simulink model "bus_roadtest_v3"  (R2018a)
settings: Solver=ode3  StartTime=0.0  StopTime=inf  FixedStep=0.01  RelTol=1e-3  EnableMultiTasking=on
PostLoadFcn:
  | , if any(exist('dsrtsu_mdlpostloadfcn', 'file') == [2, 3, 6]), try dsrtsu_mdlpostloadfcn('Execute', bdroot); catch fprintf('Error in PostLoadFcn (dsrtsu_mdlpostloadfcn) for model "%s":\n %s\n', bdroot, lasterr); end, end,
InitFcn:
  | bus_roadtest_v3_initial
values from neighbouring files (symbols this model uses):
  ay_max = 2    [Ini.m]
  delta_t = 0.01    [Ini.m]
  end_left_pass = 1    [Ini.m]
  end_right_pass = 0    [Ini.m]
  finish_node_id = length(Map_data(:,1))    [Ini.m]
  forward_length = 15    [Ini.m]
  gamma = sqrt(N_xaug+lambda)    [bus_roadtest_v3_initial.m]
  k_safe = 1    [Ini.m]
  nodes = nodes(1:index_node,:)    [Ini.m]
  rmin = 10    [Ini.m]
  segments = zeros(length(xy_ends_Pos(:,1)),3)    [Ini.m]
  start_node_id = 1    [Ini.m]
  Ts = 0.01    [bus_roadtest_v3_initial.m]
  Veh_CG = [0.5, 0.2]    [Ini.m]
  Veh_size = [1.99986,6.09558]    [Ini.m]
  vmax = 6    [Ini.m]
  weight = [weight_0,weight_0_cov,weight_i]    [bus_roadtest_v3_initial.m]
undefined symbols (not defined in the file or in its folder): Brake_table, DiscIntNeverNeededParam, Map_data, R, REF_GPS_RFS, Steer_gain_table, T
libraries: rtican x71, simulink x26, rti1401lib_adc_type4 x8, rti1401lib_dio_type4 x1
(part 15 of 18)

== matlab function bus_roadtest_v3/Positioning_module/ITRI_MM/UKF_Only/GNSS_UKF_MM ==
  data: seg_id_near output; Map_data input; dist_op output; Position_X input; op_distance output; Oi_near output; num_lane_direction output; seg_heading output; seg_LaneWidth output; Postion_Y input; Position_H input
function [seg_id_near,dist_op,op_distance,Oi_near,num_lane_direction,seg_heading,seg_LaneWidth]= fcn(Map_data,Position_X,Postion_Y,Position_H)

%%% Map_data=[Seg_XY SLOPE_SEG SHIFT_SEG Heading_X LENGTH_SEG]; nx8
XY_ID=Map_data(:,1);
XY_INI=Map_data(:,2:3);
XY_END=Map_data(:,4:5);
SLOPE_SEG=Map_data(:,6);
SHIFT_SEG=Map_data(:,7);
HEADING_DIFFERENCE_VEH_ROAD = 45*pi/180;
DIST_THREAD_5 = 4;

m=length(XY_ID);
oi_xy=zeros(m,2);
dist_op=zeros(m,1);
for i =1:m
    if SLOPE_SEG(i) == inf
        oi_xy(i,1) = XY_INI(i,1); % x position of the projection point on this segment
        oi_xy(i,2) = Postion_Y;
    elseif SLOPE_SEG(i)==0
        oi_xy(i,1) = Position_X;
        oi_xy(i,2) = XY_INI(i,2);
    else
        a_j = -1/SLOPE_SEG(i);
        b_j = Postion_Y - a_j*Position_X;
        oi_xy(i,1) = (b_j-SHIFT_SEG(i))/(SLOPE_SEG(i)-a_j); % x position of the i-th projection point
        oi_xy(i,2) = (SLOPE_SEG(i)*b_j - a_j*SHIFT_SEG(i))/(SLOPE_SEG(i)-a_j); % y position of the i-th projection point 
    end          
end

for i = 1:length(oi_xy(:,1));
    dist_op(i,1)=sqrt((oi_xy(i,1)-Position_X)^2+(oi_xy(i,2)-Postion_Y)^2);     
end

[seg_id_near,op_distance,oi_near,note,seg_direction,head_err,num_lane_direction,seg_heading] = MM(Position_H*180/pi,[Position_X;Postion_Y],oi_xy,dist_op,Map_data,HEADING_DIFFERENCE_VEH_ROAD,DIST_THREAD_5);
Oi_near=oi_near';
[~,seg_id_ind] = max(XY_ID == seg_id_near);
seg_LaneWidth = Map_data(seg_id_ind,11);
seg_Curvature = Map_data(seg_id_ind,14);

%% MM function
function [seg_id_near,op_distance,oi_near,note,seg_direction,head_err,num_lane_direction,seg_heading] = MM(heading,X_pos,oi_xy,dist_op,Map_data,HEADING_DIFFERENCE_VEH_ROAD,DIST_THREAD_5)
note=0;
seg_id_near=double(0);
op_distance=0;
oi_near=zeros(1,2);
end_pt=zeros(1,2);
seg_direction=0;
[dist_sort,index] = sort(dist_op);
index=[index,zeros(length(index),1)];

xy_ini = Map_data(:,2:3);
xy_end = Map_data(:,4:5);
SLOPE_SEG = Map_data(:,6);
seg_id = Map_data(:,1);
LENGTH_SEG = Map_data(:,9);
SEG_GPS_HEAD = Map_data(:,8);
SEG_GPS_HEAD=[seg_id SEG_GPS_HEAD];

%%    Map Matching

for j = 1:length(xy_ini(:,1));
    i = index(j,1);
    dis_temp1 = sqrt((xy_ini(i,1)-oi_xy(i,1))^2+(xy_ini(i,2)-oi_xy(i,2))^2);
    dis_temp2 = sqrt((xy_end(i,1)-oi_xy(i,1))^2+(xy_end(i,2)-oi_xy(i,2))^2);
 
    if (dis_temp1 <= LENGTH_SEG(i)&& dis_temp2 <= LENGTH_SEG(i));
        index(j,2) = 1; %oi_xy lies in between xy_ini and xy_end
    else index(j,2) = 0;
    end
end

%"possible_seg" contains the sequence of possible segment index
ind_temp = find(index(1:end,2)==1);
% ind_temp=ind_temp(1);
if isempty(ind_temp);
   note = 1;  % 1: the projection point is not between two segment ends for any road segment;
              % search nearest segment by finding the nearest segment end!             
   %compare distances between ends and X_pos!     
    dist_ini = rel_dist_xy(X_pos,xy_ini);
    dist_end = rel_dist_xy(X_pos,xy_end);
  
    [min_dis_ini,junk1] = min(dist_ini);   %-------------------------------------------------哪來的junk 1 &2 ?
    [min_dis_end,junk2] = min(dist_end);
    if min_dis_ini<= min_dis_end; %X_pos is closer to the end
       possible_seg = junk1; %index
       end_pt = xy_ini(junk1,1:end);
    else 
       possible_seg = junk2; %index
       end_pt = xy_end(junk2,1:end);
    end

    seg_id_near = seg_id(possible_seg);
    
    op_distance = dist_op(possible_seg);
    oi_near = oi_xy(possible_seg,1:2);
    if possible_seg>1 && possible_seg<length(seg_id)
    op_distance_n=rel_dist_xy(X_pos,oi_near);
    min_ini_pos=rel_dist_xy(X_pos,xy_ini(possible_seg,:));
    min_end_pos=rel_dist_xy(X_pos,xy_end(possible_seg,:));
    if op_distance_n<min_ini_pos && op_distance_n<min_end_pos
        note = 0;
    else
        note = 1;
    end
    else
        op_distance_n=rel_dist_xy(X_pos,oi_near);
        min_ini_pos=rel_dist_xy(X_pos,xy_ini(possible_seg,:));
        min_end_pos=rel_dist_xy(X_pos,xy_end(possible_seg,:));
    end
    
%    seg_direction = Get_Seg_Heading(seg_id_near,heading);
%    %%%不用老師程式--
    temp_ind = find(SEG_GPS_HEAD(:,1) == seg_id_near);
    head_err = abs(heading-SEG_GPS_HEAD(temp_ind(1),2)); 
    if head_err <= HEADING_DIFFERENCE_VEH_ROAD
    seg_direction = 1; %1= along slope, 2:adverse
    elseif head_err>=HEADING_DIFFERENCE_VEH_ROAD && head_err<=90
    seg_direction = 0; %unknown
    else
    seg_direction = 2;
    end
%     %%%不用老師程式--
 elseif length(ind_temp(1)) ==1; %only 
%      find one segment candidate
       note = 0; % 0: the projection point lies between two ends of each segment    
       possible_seg = index(ind_temp(1),1);
       seg_id_near = seg_id(possible_seg);
       op_distance = dist_op(possible_seg);
       oi_near = oi_xy(possible_seg,1:2);
       end_pt = [0,0]; % temp./unused nominal values
%      seg_direction = Get_Seg_Heading(seg_id_near,heading); %get road segment heading direction

        temp_ind = find(SEG_GPS_HEAD(:,1) == seg_id_near);
        head_err = abs(heading-SEG_GPS_HEAD(temp_ind(1),2)); 
       if head_err <= HEADING_DIFFERENCE_VEH_ROAD;
            seg_direction = 1; %1= along slope, 2:adverse
       elseif head_err>=HEADING_DIFFERENCE_VEH_ROAD && head_err<=90
            seg_direction = 0; %unknown
       else
            seg_direction = 2;
       end
       %Now compare the distances between X_pos and all segment ends with
       %op_distance. If find closer node, may discard previous found segment.
       
       dist_ini = rel_dist_xy(X_pos,xy_ini);
       dist_end = rel_dist_xy(X_pos,xy_end);
           %dis_min = min(dist_ini,dist_end);
           %dis_min_val = min(dis_min);
           %temp_a = find(dis_min == dis_min_val); % diff, segments may have the same node!
       [min_dis_ini,junk1] = min(dist_ini);
       [min_dis_end,junk2] = min(dist_end);
       dis_min_val = min(min_dis_ini,min_dis_end);
       
    if dis_min_val < op_distance;%min(op_distance); %X_pos is closer to one of the segment ends than its project point         
       note = 2; %Change the "note" value! 
                 %special case: the found projection pt. (oi_near) lie(s) between two ends 
                 %of one segment, but the associated segments may not
                 %the nearest road segments.          
       %search the nearest node of road segments. 
        if min_dis_ini<= min_dis_end;
           temp_a = junk1;
           end_pt = xy_ini(junk1,1:end);
        else 
           temp_a = junk2;
           end_pt = xy_end(junk2,1:end);
        end
       
        
        if length(temp_a)>1; %multiple segment case
            
           seg_head_pos = SEG_GPS_HEAD(temp_a,2); %road segment heading in the positive slope direction
%            seg_head_neg = SEG_GPS_HEAD(temp_a,3);
           
           %find smallest heading discrepancy in positive slope direction
           [junk1,ind_pos] = min(abs(heading - seg_head_pos(1:end)));
               
           %find smallest heading discrepancy in negative/adverse slope direction
%            [junk2,ind_neg] = min(abs(angle_convert(heading - seg_head_neg(1:end))));
           
           %compare two smallest heading erros of two adverse directions
 
              ind = temp_a(ind_pos);
              seg_id_near = seg_id(ind);
              op_distance = dist_op(ind);
              oi_near = oi_xy(ind,1:2);
              temp_ind = find(SEG_GPS_HEAD(:,1) == seg_id_near);
              head_err = abs(heading-SEG_GPS_HEAD(temp_ind(1),2)); 

              if head_err <= HEADING_DIFFERENCE_VEH_ROAD;
                    seg_direction = 1; %1= along slope, 2:adverse
              elseif head_err>=HEADING_DIFFERENCE_VEH_ROAD && head_err<=90
                    seg_direction = 0; %unknown
              else
                    seg_direction = 2;
              end
       
        else %single segment case
              temp_ind = find(SEG_GPS_HEAD(:,1) == seg_id_near);
              head_err = abs(heading-SEG_GPS_HEAD(temp_ind(1),2)); 

              if head_err <= HEADING_DIFFERENCE_VEH_ROAD;
                    seg_direction = 1; %1= along slope, 2:adverse
              elseif head_err>=HEADING_DIFFERENCE_VEH_ROAD && head_err<=90
                    seg_direction = 0; %unknown
              else
                    seg_direction = 2;
              end
                 seg_id_near = seg_id(temp_a);
                 op_distance = dist_op(temp_a);
                 oi_near = oi_xy(temp_a,1:2);
        end
    end
 else %multiple segment candidates
       note = 0; % 0: the projection point lies between two ends of each segment          
       cand_seg = index(ind_temp,1);
       %cand_id = seg_id(cand_seg(1:2)); % only check the first two colsest segment candidate
       cand_op_dist = dist_op(cand_seg(1:2));
       
       %find road heading for the first two candidates
        head_pos = SEG_GPS_HEAD(cand_seg(1:2),2);

       %first candidate
        err_1 =  abs(heading - head_pos(1));
        %temp = [head_pos(1),head_neg(1)];
        %cand_head(1) = temp(ii);
        %clear ii;
       %second candidate
        err_2 = abs(heading - head_pos(2));
        %temp = [head_pos(2),head_neg(2)];
        %cand_head(2) = temp(ii);
        %clear ii;
        
       %compare two heading errors
        if err_1<= err_2 && err_1< HEADING_DIFFERENCE_VEH_ROAD; % HEADING_DIFFERENCE_VEH_ROAD = 45/180*pi
           possible_seg =  cand_seg(1);
           seg_direction = 1;
        elseif err_2< err_1 && ((cand_op_dist(2)-cand_op_dist(1))< DIST_THREAD_5); %DIST_THREAD_5 = 9 m
           possible_seg = cand_seg(2); 
           seg_direction = 2;
        else
           possible_seg = cand_seg(1);
           seg_direction = 1;
        end
        
       clear err_1 err_2 cand_op_dist cand_seg head_pos head_neg direction_1 direction_2;
       %possible_seg = index(ind_temp,1);       
       seg_id_near = seg_id(possible_seg);
       op_distance = dist_op(possible_seg);
       oi_near = oi_xy(possible_seg,1:2);
       end_pt = [0,0]; % temp./unused nominal values
        
       %Now compare the distances between X_pos and all segment ends with
       %above op_distance.
       %compute distances between X_pos and all segment ends
       dist_ini = rel_dist_xy(X_pos,xy_ini);
       dist_end = rel_dist_xy(X_pos,xy_end);
           %dis_min = min(dist_ini,dist_end);
           %dis_min_val = min(dis_min);
           %temp_a = find(dis_min == dis_min_val); % diff, segments may have the same node!
       [min_dis_ini,junk1] = min(dist_ini);
       [min_dis_end,junk2] = min(dist_end);
       dis_min_val = min(min_dis_ini,min_dis_end); 
       
    if dis_min_val < op_distance; %min(op_distance); %X_pos is closer to one of the segment ends than its project point         
       note = 2; %Change the note value! 
                 %special case: the found projection pt. (oi_near) lie(s) between two ends 
                 %of one segment, but the associated segments may not be
                 %the nearest road segments.          
       %search the nearest node of road segments. 
        if min_dis_ini<= min_dis_end;
           temp_a = junk1;
           end_pt = xy_ini(junk1,1:2);
        else 
           temp_a = junk2;
           end_pt = xy_end(junk2,1:2);
        end
        clear junk1 junk2;
        
        if length(temp_a)>1; %multiple segment case, then compare heading with road segment heading
          
           seg_head_pos = SEG_GPS_HEAD(temp_a,2);
           [junk1,ind_pos] = min(abs(heading - seg_head_pos(1:end)));


              ind = temp_a(ind_pos);
              seg_id_near = seg_id(ind);
              op_distance = dist_op(ind);
              oi_near = oi_xy(ind,1:2);

              temp_ind = find(SEG_GPS_HEAD(:,1) == seg_id_near);
              head_err = abs(heading-SEG_GPS_HEAD(temp_ind(1),2)); 

              if head_err <= HEADING_DIFFERENCE_VEH_ROAD;
                    seg_direction = 1; %1= along slope, 2:adverse
              elseif head_err>=HEADING_DIFFERENCE_VEH_ROAD && head_err<=90
                    seg_direction = 0; %unknown
              else
                    seg_direction = 2;
              end

       
        else %determine road direction is positive or negative slope direction

             seg_id_near = seg_id(temp_a);
             op_distance = dist_op(temp_a);
             oi_near = oi_xy(temp_a,1:2);
             temp_ind = find(SEG_GPS_HEAD(:,1) == seg_id_near);
              head_err = abs(heading-SEG_GPS_HEAD(temp_ind(1),2)); 

              if head_err <= HEADING_DIFFERENCE_VEH_ROAD;
                    seg_direction = 1; %1= along slope, 2:adverse
              elseif head_err>=HEADING_DIFFERENCE_VEH_ROAD && head_err<=90
                    seg_direction = 0; %unknown
              else
                    seg_direction = 2;
              end

        end
    end
           
end
%% check projection distance positive or negative Y=AX+B ;AX+B-Y>0 or AX+B-Y<0
Heading_X_rad = Map_data(:,8).*pi./180;
[~,temp_ind] = max(seg_id(:,1) == seg_id_near);
A=SLOPE_SEG(temp_ind);
B=oi_near(2)-A*oi_near(1);
if A < 0
    C=-A*X_pos(1)-B+X_pos(2);
    if Heading_X_rad(temp_ind) > 3*pi/2 && Heading_X_rad(temp_ind) < 2*pi
        C = C;
    else
        C = -C;
    end
elseif A == 0
    if oi_near(2)<X_pos(2)
        C=-1;
    else
        C=1;
    end
else
    C=A*X_pos(1)+B-X_pos(2);
    if Heading_X_rad(temp_ind) > pi && Heading_X_rad(temp_ind) < 3*pi/2
        C = C;
    else
        C = -C;
    end
end
if C<0 
    d=1;
elseif C==0
    d=1;
else
    d=-1;
end
num_lane_direction=[A;B;C;d];
seg_heading = Heading_X_rad(temp_ind);
%% rel_dist
function dist = rel_dist_xy(ref_xy,pt_xy)
% This function computes relative distances between given reference point, ref_xy, and positions, p_xy. 
% ref_xy = [x0,y0];
% pt_xy = [x,y];

temp = (pt_xy(:,1)-ref_xy(1)).^2 + (pt_xy(:,2)-ref_xy(2)).^2;
dist = temp.^0.5;

== matlab function bus_roadtest_v3/Target_planner/MATLAB Function1 ==
  data: ID input; Path_flag output; switch_flag input
function Path_flag = fcn(ID,switch_flag)

% if switch_flag == 1
%     if ID >= 187 || ID <= 3
%         Path_flag = 1;
%     else
%         Path_flag = 0;
%     end
% else
    Path_flag = 0;
% end

== matlab function bus_roadtest_v3/Flag_management/Fault detection/Fault detection(Control)/RSU fault detection ==
  data: V2X_Phase input; V2X_Remaintime input; RSU_fault output; Light_Distance input
function RSU_fault  = fcn(V2X_Phase,V2X_Remaintime,Light_Distance)

RSU_fault  = 0;
if Light_Distance<50 && ((V2X_Phase==0&&V2X_Remaintime~=-0.1) && V2X_Phase~=1 && V2X_Phase~=2 && V2X_Phase~=3)
    RSU_fault = 1;
end

== matlab function bus_roadtest_v3/Target_planner/target_seg_id_search ==
  data: Static_Path_0 input size=size(Map_data); Forward_Static_Path_x output size=length(nodes(:,1)); Vehicle_state input; SEG_ID_NEAR_TRUE input; Car_Velocity input; LAT input; Forward_Static_Path_y output size=length(nodes(:,1)); Forward_Static_Path_id output size=length(nodes(:,1)); start_ind_out output; seg_id output size=size(Map_data(:,1)); end_seg_id output; case_0 output; end_ind output; LAS0 input
function [Forward_Static_Path_x,Forward_Static_Path_y,Forward_Static_Path_id,start_ind_out,seg_id,end_seg_id,case_0,end_ind]= FowardSeg(Static_Path_0,Vehicle_state,SEG_ID_NEAR_TRUE,Car_Velocity,LAT,LAS0)

forward_length = Car_Velocity*LAT+LAS0;

Static_Path = Static_Path_0;

x = Vehicle_state(1,1); %vehicle global coordinate
y = Vehicle_state(2,1);

xy_ends_POS = Static_Path(:,2:5);
seg_id = Static_Path(:,1);
seg_length = Static_Path(:,9);

if xy_ends_POS(1,1) == xy_ends_POS(end,3) && xy_ends_POS(1,2) == xy_ends_POS(end,4)
    Static_PathCycle = 1;
else
    Static_PathCycle = 0;
end

[~,start_ind] = max(seg_id(:) == SEG_ID_NEAR_TRUE);
% start_ind = find(seg_id(:) == SEG_ID_NEAR_TRUE);
start_ind_out = start_ind(1);
% 加入從長度判定要幾個seg 預計至少20m
total_length = ((x-xy_ends_POS(start_ind(1),3))^2+(y-xy_ends_POS(start_ind(1),4))^2)^0.5;
end_ind_0 = start_ind(1);
case_0 = 0;
end_ind = 0;
for i = 1 : length(seg_length)
    if total_length > forward_length
        end_ind = end_ind_0;
        break;
    end
    if (start_ind(1)+i) <= length(seg_length)
        total_length = total_length + seg_length(start_ind(1)+i);
        end_ind_0 = start_ind(1)+i;
        case_0 = 1;
    else
        if Static_PathCycle == 1
            total_length = total_length + seg_length(start_ind(1)+i-length(seg_length));
            end_ind_0 = start_ind(1)+i - length(seg_length);
            case_0 = 2;
        else
            total_length = total_length;
            end_ind = end_ind_0;
            case_0 = 3;
            break;
        end
    end
end

Forward_Static_Path_id_0 = zeros(length(seg_id),1);
if isempty(start_ind) == 1
    start_ind(1) = 1;
    end_ind = length(seg_id(:));
    Static_Path_ends_POS = xy_ends_POS(start_ind(1):end_ind(1),:);
    Forward_Static_Path_id_0(:) = seg_id(:);
    Forward_Static_Path_length = length(seg_id(:));
else
    if case_0 == 1 || case_0 == 0
        Static_Path_ends_POS = xy_ends_POS(start_ind(1):end_ind(1),:);
        Forward_Static_Path_id_0(1:(end_ind(1)-start_ind(1)+1)) = seg_id(start_ind(1):end_ind(1));
        Forward_Static_Path_length = length(seg_id(start_ind(1):end_ind(1)));
    else
        if case_0 == 2
            Static_Path_ends_POS = [xy_ends_POS(start_ind(1):end,:);xy_ends_POS(1:end_ind(1),:)];
            Forward_Static_Path_id_0(1:(1+length(seg_id(:))-start_ind(1)+end_ind(1))) = [seg_id(start_ind(1):end);seg_id(1:end_ind(1))];
            Forward_Static_Path_length = length([seg_id(start_ind(1):end);seg_id(1:end_ind(1))]);
        else
            end_ind = length(seg_id(:));
            Static_Path_ends_POS = xy_ends_POS(start_ind(1):end_ind(1),:);
            Forward_Static_Path_id_0(1:end_ind(1)-start_ind(1)+1) = seg_id(start_ind(1):end_ind(1));
            Forward_Static_Path_length = length(seg_id(start_ind(1):end_ind(1)));
        end
    end
end

Forward_Static_Path_id = Forward_Static_Path_id_0(1:Forward_Static_Path_length);

Forward_Static_Path = zeros(length(Static_Path_ends_POS(:,1))+1,2);
Forward_Static_Path(1:length(Static_Path_ends_POS(:,1)),1:2) = Static_Path_ends_POS(:,1:2);
Forward_Static_Path(length(Static_Path_ends_POS(:,1))+1,1:2) = Static_Path_ends_POS(length(Static_Path_ends_POS(:,1)),3:4);

Forward_Static_Path_x = Forward_Static_Path(1:numel(Forward_Static_Path(:,1)),1);
Forward_Static_Path_y = Forward_Static_Path(1:numel(Forward_Static_Path(:,1)),2);

end_seg_id = Forward_Static_Path_id(end);

% Forward_Static_Path_id = seg_id(start_ind_out:end);
% Forward_Static_Path_x = [xy_ends_POS(start_ind_out:end,1);xy_ends_POS(end,3)];
% Forward_Static_Path_y = [xy_ends_POS(start_ind_out:end,2);xy_ends_POS(end,4)];

== matlab function bus_roadtest_v3/Positioning_module/ITRI_MM/UKF_Only/GNSS_Check/WithoutRTK ==
  data: GPS_X input; GPS_update output; GPS_Y input; GPS_Heading input; Road_Alt_GPS input; IMU_Sensor input; GPS_TYPE input; X_UKF input; GPS_X_Acc input; GPS_Y_Acc input; Q_last_i input; R_last_i input; Last_GPS_In input; X_state output; GNSS_FaultFlag output; Q_last_o output; R_last_o output; Last_GPS_Out output
function [GPS_update,X_state,GNSS_FaultFlag,Q_last_o,R_last_o,Last_GPS_Out] = fcn(GPS_X,GPS_Y,GPS_Heading,Road_Alt_GPS,IMU_Sensor,GPS_TYPE,X_UKF,GPS_X_Acc,GPS_Y_Acc,Q_last_i,R_last_i,Last_GPS_In)

Last_X=Last_GPS_In(1);
Last_Y=Last_GPS_In(2);
Last_Heading = Last_GPS_In(3);
Sensor_Velocity = IMU_Sensor(1);
Sensor_Yawrate=IMU_Sensor(2);
Sensor_Grade=IMU_Sensor(3);

dist_gpslastgps = sqrt((GPS_X-X_UKF(1))^2 + (GPS_Y-X_UKF(2))^2);
if dist_gpslastgps > 10
    GNSS_FaultFlag = 1;
else
    GNSS_FaultFlag = 0;
end
if GPS_X==Last_X && GPS_Y==Last_Y
    GPS_update = 0;
else
    if Sensor_Velocity >= 0.1 && dist_gpslastgps > 10
        GPS_update = 0;
    else
        GPS_update = 1;
    end
end

if Sensor_Velocity >= 0.1
    if dist_gpslastgps > 10
        GPS_X_out = Last_X;
        GPS_Y_out = Last_Y;
        GPS_Heading_out = Last_Heading;
        Q = Q_last_i;
        R = R_last_i;
    else
        GPS_X_out = GPS_X;
        GPS_Y_out = GPS_Y;
        GPS_Heading_out = GPS_Heading;
        Q = diag([0.0001,0.0001,0.000001,1,0.0001]);
        R = diag([GPS_X_Acc,GPS_Y_Acc,5,0.05,0.0001]);
    end
else
    GPS_X_out = GPS_X;
    GPS_Y_out = GPS_Y;
    GPS_Heading_out = GPS_Heading;
    Q = diag([0.0001,0.0001,0.000001,1,0.0001]);
    R = diag([5,5,5,0.05,0.0001]);
end

Q_last_o = Q;
R_last_o = R;

Last_GPS_Out = [GPS_X_out;GPS_Y_out;GPS_Heading_out];
X_state = [GPS_X_out,GPS_Y_out,GPS_Heading_out,Sensor_Yawrate,Sensor_Velocity]';

== matlab function bus_roadtest_v3/Positioning_module/ITRI_MM/UKF_Only/MATLAB Function ==
  data: Map_data input size=size(Map_data(:,:)); forward_path output; seg_id_near input; forward_segid output
function [forward_path,forward_segid] = fcn(Map_data,seg_id_near)

forward_path = [Map_data(end,:);Map_data(end,:);Map_data(end,:);Map_data(end,:);Map_data(end,:)];

[~,seg_start_ind] = max(Map_data(:,1) == seg_id_near);

if seg_start_ind + 4 <= length(Map_data(:,1))
    seg_end_ind = seg_start_ind + 4;
else
    seg_end_ind = length(Map_data(:,1));
end

index = 0;
for i = seg_start_ind : seg_end_ind
    index = index + 1;
    forward_path(index,:) = Map_data(i,:);
end

forward_segid = forward_path(:,1);

== matlab function bus_roadtest_v3/Flag_management/State toggle ==
  settings: updateMethod=DISCRETE
  data: Drive_start input; Self_driving_on output; Drive_stop input; Static_flag input; AEB_flag input; Idle_flag input
function Self_driving_on = fcn(Drive_start,Drive_stop,Static_flag,AEB_flag,Idle_flag)

persistent State Stop_trig;
if isempty(State)
    State = 0;
    Stop_trig = 0;
end 

% Drive start button activated
if (Drive_start ==1 && State == 0)
    State = 1;
    Stop_trig = 0;
end

% Drive stop button activated
if (Drive_stop ==1 && State == 1)
    Stop_trig = 1;
    State = 1;
end

% Vehicle fully stops
if (Static_flag ==1 && Stop_trig ==1)
    State = 0;
end

% AEB trigger
if (AEB_flag == 1) || (Idle_flag == 1)
    Stop_trig = 1;
    State = 0;
end

Self_driving_on = State;

== matlab function bus_roadtest_v3/Target_planner/Steer_gain_scheduling ==
  data: Look_ahead_time output; U_turn input; Look_ahead_S0 output; Steer_gain_table input; K_gain output
function [Look_ahead_time,Look_ahead_S0,K_gain] = fcn(U_turn,Steer_gain_table)

% Steer_gain_table format
% [S0,look_ahead_time,K_gain;   (LKC_gain)
%  S0,look_ahead_time,K_gain;]  (U_turn gain)

% Road geometry assessment



% Gain scheduling

if (U_turn == 1)
    Look_ahead_S0 = Steer_gain_table(2,1);
    Look_ahead_time = Steer_gain_table(2,2);
    K_gain = Steer_gain_table(2,3);
else
    Look_ahead_S0 = Steer_gain_table(1,1);
    Look_ahead_time = Steer_gain_table(1,2);
    K_gain = Steer_gain_table(1,3);
end

== matlab function bus_roadtest_v3/Flag_management/MATLAB Function ==
  settings: updateMethod=DISCRETE
  data: Drive_start_button input; Drive_stop_button input; TouchP_start input; TouchP_start_RX input; System_ready input; Drive_start output; Drive_stop output; Actual_state input; Drive_state_out output
function [Drive_start, Drive_stop, Drive_state_out] = fcn(Drive_start_button, Drive_stop_button, TouchP_start,TouchP_start_RX, System_ready, Actual_state)
persistent Drive_state;
if isempty(Drive_state)
    Drive_state = 0;
end 
Drive_start = 0;
Drive_stop = 0;
if Drive_start_button==1
    Drive_state = 1;
end
if Drive_stop_button==1
    Drive_state = 0;
end
if TouchP_start==1 && TouchP_start_RX ==1 && Drive_state==0 
    Drive_start = 1;
    Drive_state = 1;
end
if TouchP_start==0 && TouchP_start_RX ==1 && Drive_state==1 
    Drive_stop = 1;
    Drive_state = 0;
end
if System_ready==0 && Drive_state==1 
    Drive_stop = 1;
    Drive_state = 0;
end
Drive_state_out = Drive_state;

== matlab function bus_roadtest_v3/Motion_controller/Longitudinal_control/Switching_module/Brake_status ==
  data: AEB input; Brake_status output; Static input; CC_trig input; interrupt input
function Brake_status = Brake_status(AEB,Static,CC_trig,interrupt)

if (interrupt == 1)
    Brake_status = 4;
elseif (AEB ==1)
    Brake_status = 3;
elseif (Static == 1)
    Brake_status = 2;
elseif (CC_trig ==1)
    Brake_status = 1;
else
    Brake_status = 0;
end

== matlab function bus_roadtest_v3/Data_RX/Xavier/MATLAB Function13 ==
  data: Radar_speed input; Radar_speed_out output; Radar_distance input; Radar_RX input; Radar_speed_pre input; Radar_distance_pre input; Radar_distance_out output; time_out output
function [Radar_speed_out, Radar_distance_out, time_out] = fcn(Radar_speed, Radar_distance,Radar_RX, Radar_speed_pre, Radar_distance_pre)

persistent count;
persistent time;

if isempty(count)
    count = 0;
    time = 0;
end 

if ((Radar_distance-Radar_distance_pre)>15) && (count<10)
    Radar_speed_out = Radar_speed_pre;
    Radar_distance_out = Radar_distance_pre;
    count = count + 1;
else
    if Radar_speed>10
        Radar_speed_out = 10;
    elseif Radar_speed<-10
        Radar_speed_out = -10;
    else
        Radar_speed_out = Radar_speed;
    end  
    Radar_distance_out = Radar_distance;
    count = 0;
end

if (Radar_RX == 1)
    time = 0;
else
    time = time + 1;
end
if (time>50)
    Radar_distance_out = 80;
    Radar_speed_out = 0;
end
time_out = time;

== matlab function bus_roadtest_v3/Positioning_module/ITRI_MM/UKF_Only/GNSS_Check/Multipath_detection ==
  data: GPS_X input; GPS_update_True output; GPS_Y input; X_UKF input; GPS_X_Acc input; GPS_Y_Acc input; Last_GPS_In input; GNSS_FaultFlag_True output; Last_GPS_Out output; Last_UKF_Out output; Last_GPS_est_Out output; Last_UKF_In input; Last_GPS_est_In input; count_i input; count_o output
function [GPS_update_True,GNSS_FaultFlag_True,Last_GPS_Out,Last_UKF_Out,Last_GPS_est_Out,count_o] = fcn(GPS_X,GPS_Y,X_UKF,GPS_X_Acc,GPS_Y_Acc,Last_GPS_In,Last_UKF_In,Last_GPS_est_In,count_i)
GNSS_FaultFlag_True = 0;

Last_X=Last_GPS_In(1);
Last_Y=Last_GPS_In(2);

Last_UKF_X = Last_UKF_In(1);
Last_UKF_Y = Last_UKF_In(2);
X_UKF_X = X_UKF(1);
X_UKF_Y = X_UKF(2);
Last_GPS_X_est = Last_GPS_est_In(1);
Last_GPS_Y_est = Last_GPS_est_In(2);

if GPS_X==Last_X && GPS_Y==Last_Y
    GPS_update_True = 0;
    count_o = count_i + 1;
else
    count_o = 0;
    GPS_update_True = 1;
end

if GPS_update_True == 1
    GPS_X_err = GPS_X - (Last_GPS_X_est + X_UKF_X - Last_UKF_X);
    GPS_Y_err = GPS_Y - (Last_GPS_Y_est + X_UKF_Y - Last_UKF_Y);
    GPS_err = sqrt(GPS_X_err^2 + GPS_Y_err^2);
    if GPS_err > 10
        GNSS_FaultFlag_True = 1;
    end
    GPS_X_est_out = GPS_X;
    GPS_Y_est_out = GPS_Y;
else
    if count_o >= 100
        GNSS_FaultFlag_True = 1;
    end
    GPS_X_est_out = Last_GPS_X_est + X_UKF_X - Last_UKF_X;
    GPS_Y_est_out = Last_GPS_Y_est + X_UKF_Y - Last_UKF_Y;
end
    
GPS_X_out = GPS_X;
GPS_Y_out = GPS_Y;
X_UKF_X_out = X_UKF_X;
X_UKF_Y_out = X_UKF_Y;

Last_GPS_Out = [GPS_X_out;GPS_Y_out];
Last_UKF_Out = [X_UKF_X_out;X_UKF_Y_out];
Last_GPS_est_Out = [GPS_X_est_out;GPS_Y_est_out];

== matlab function bus_roadtest_v3/Flag_management/State management/bus_stop_statemachine ==
  settings: updateMethod=DISCRETE
  data: SLAM_seg_id input; Stop_Mission output; Static_flag input; Bus_state_forstop output
function [Stop_Mission, Bus_state_forstop] = fcn(SLAM_seg_id, Static_flag)
% Mission -> next stop
% Bus_state_forstop -> 0=Crusing, 1=incoming, 2=stopping, 3=leaving
persistent Bus_status
if isempty(Bus_status)
    Bus_status = 0;
end 

Stop_zone = 0;
Stop_Mission = 99;
if SLAM_seg_id>=1 && SLAM_seg_id<30
    Stop_Mission = 1;
    Stop_zone = 1;
elseif SLAM_seg_id>=999 && SLAM_seg_id<999
    Stop_Mission = 2;
    Stop_zone = 1;
end

% if SLAM_seg_id>=1 && SLAM_seg_id<4
%     Stop_Mission = 1;
%     Stop_zone = 1;
% elseif SLAM_seg_id>=90 && SLAM_seg_id<94 
%     Stop_Mission = 2;
%     Stop_zone = 1;
% elseif SLAM_seg_id>=165 && SLAM_seg_id<168 
%     Stop_Mission = 3;
%     Stop_zone = 1;
% elseif SLAM_seg_id>=245 && SLAM_seg_id<253 
%     Stop_Mission = 4;
%     Stop_zone = 1;
% elseif SLAM_seg_id>=280 && SLAM_seg_id<290
%     Stop_Mission = 5;
%     Stop_zone = 1;
% end

if Bus_status==0 && Stop_zone==1
    Bus_status = 1;
end
if Bus_status==1 && Static_flag==1
    Bus_status = 2;
end
if Bus_status==2 && Static_flag==0
    Bus_status = 3;
end
if Stop_zone==0
    Bus_status = 0;
end
Bus_state_forstop = Bus_status;

== matlab function bus_roadtest_v3/Data_RX/X-by-wire/Brake/MATLAB Function ==
  settings: updateMethod=DISCRETE
  data: Brake_trig input; brake_trig_last input; Brake_interrupt output; Pressure_cmd input; Pressure_fb input; Brake_release output; Release_time input
function [Brake_interrupt,Brake_release] = fcn(Brake_trig,brake_trig_last,Pressure_cmd,Pressure_fb,Release_time)

% Use Record 328
persistent brake_release counter 
if isempty(brake_release)
    brake_release = 0;
    counter = 0;
end 

% State check
if brake_trig_last > 0
    if Brake_trig == 0
        brake_release = 1;
    end
end

if brake_release == 1
    if Brake_trig == 1
        brake_release = 0;
        counter = 0;
    else
        if counter < Release_time
            counter = counter +1;
        else
            brake_release = 0;
            counter = 0;
        end
    end
end

% Interrupt check
if Pressure_cmd==0 && Pressure_fb>=0.4 && brake_release == 0
    Brake_interrupt = 1;
else
    Brake_interrupt = 0;
end

Brake_release = brake_release;

== matlab function bus_roadtest_v3/Flag_management/State management/Light_state_camera  ==
  settings: updateMethod=DISCRETE
  data: SLAM_seg_id_near input; color_light input; Light_info_out output; direction_light input
function Light_info_out = fcn(SLAM_seg_id_near,color_light,direction_light)
% color_light 0=unknown, 1=red, 2=yellow, 3=green
% output light info 0=no message, 1=red, 2=green,3=yellow

persistent Light_info;
if isempty(Light_info)
    Light_info = 0;
end 

if SLAM_seg_id_near>=114 && SLAM_seg_id_near<134
    if color_light==1 || color_light==2 
        Light_info =1;
    elseif color_light==3 || direction_light~=0
        Light_info =2;
    elseif color_light==0
        Light_info =0;
    end
elseif SLAM_seg_id_near>=134 && SLAM_seg_id_near<154
    if color_light==1 || color_light==2 
        Light_info =1;
    elseif color_light==3 || direction_light~=0
        Light_info =2;
    elseif color_light==0
        Light_info =0;
    end
elseif SLAM_seg_id_near>=218 && SLAM_seg_id_near<238
    if color_light==1 || color_light==2 
        Light_info =1;
    elseif color_light==3 || direction_light~=0
        Light_info =2;
    elseif color_light==0
        Light_info =0;
    end
elseif SLAM_seg_id_near>=238 && SLAM_seg_id_near<252
    if color_light==1 || color_light==2 
        Light_info =1;
    elseif color_light==3 || direction_light~=0
        Light_info =2;
    elseif color_light==0
        Light_info =0;
    end
elseif SLAM_seg_id_near>=252 && SLAM_seg_id_near<267
    if color_light==1 || color_light==2 
        Light_info =1;
    elseif color_light==3 || direction_light~=0
        Light_info =2;
    elseif color_light==0
        Light_info =0;
    end
elseif SLAM_seg_id_near>=309 && SLAM_seg_id_near<329
    if color_light==1 || color_light==2 
        Light_info =1;
    elseif color_light==3 || direction_light~=0
        Light_info =2;
    elseif color_light==0
        Light_info =0;
    end
else
    Light_info =0;
end

Light_info_out = Light_info;

== matlab function bus_roadtest_v3/Positioning_module/ITRI_MM/UKF_Only/GNSS_UKF ==
  data: Q input; R input; X output; X_AUG input; X_state input; IMU_Sensor input; Sensor_dt input; GNSS_update input; weighting input; P output; K output; x_aug output; d_GC input
function [X,P,K,x_aug] = fcn(Q,R,X_AUG,X_state,IMU_Sensor,Sensor_dt,GNSS_update,weighting,d_GC)
%#codegen

%% parameters setup

%%% X_State=[X,Y,Heading]
x_aug=X_AUG(:,1:11);
vx=IMU_Sensor(1)*1;
wz=IMU_Sensor(2);
Grade=IMU_Sensor(3);
dt=Sensor_dt;
weight_0=weighting(1);
weight_0_cov=weighting(2);
weight_i=weighting(3);
X=zeros(5,1);
N=5;

%%
%%% model 1 : slope detection
    x_aug(1,:) = x_aug(1,:) + (dt*x_aug(5,:)).*cos(x_aug(3,:)) + dt.*wz*d_GC*cos(x_aug(3,:)+pi/2); %north
    x_aug(2,:) = x_aug(2,:) + (dt*x_aug(5,:)).*sin(x_aug(3,:)) + dt.*wz*d_GC*sin(x_aug(3,:)+pi/2);%east
    x_aug(3,:) = x_aug(3,:) + (dt.*x_aug(4,:));                  %heading (radian)
    x_aug(4,:) = x_aug(4,:);
    x_aug(5,:) = x_aug(5,:);
    

 %% state process

X(1,1) = x_aug(1,1)*weight_0 + sum(x_aug(1,2:end))*weight_i;
X(2,1) = x_aug(2,1)*weight_0 + sum(x_aug(2,2:end))*weight_i;
X(3,1) = x_aug(3,1)*weight_0 + sum(x_aug(3,2:end))*weight_i;
X(4,1) = x_aug(4,1)*weight_0 + sum(x_aug(4,2:end))*weight_i;
X(5,1) = x_aug(5,1)*weight_0 + sum(x_aug(5,2:end))*weight_i;
% X = X*10^6;

    P = weight_0_cov.*((x_aug(1:5,1)-X(1:5,1))*(x_aug(1:5,1)-X(1:5,1))');

for i = 2:(2*N+1)
    
    P = P + weight_i.*((x_aug(1:5,i)-X(1:5,1))*(x_aug(1:5,i)-X(1:5,1))');

end
% P = P*10^6;

P = P + Q;

if X(3,1) < 0
    X(3,1) = X(3,1) + 2*pi;
elseif X(3,1) >= 2*pi
    X(3,1) = X(3,1) - 2*pi;
else
    X(3,1) = X(3,1);
end
%% kalman filter
if GNSS_update >0 %close-loop
    
 
        Z = X_state;

        Z_e = X; %=H*X; % observation estimate using a-priori state estimate
   %K = P*H'*inv(H*P*H'+R); % Kalman gain
        K = P*inv(P+R); %H = eye(3) %K = P*inv(P+R)
   %X = X + K*(Z - Z_e); % a-posteriori state estimate
        dZ = Z - Z_e;
        X = X + K*dZ; % a-posteriori state estimate
   
   %P = (eye(3) - K*H)*P;
  
   
        P = (eye(5) - K)*P;

        
else %open loop
        
        K = zeros(5,5);
        Z = X_state([4,5]); 
        Z_e = X([4,5]); %=H*X; % observation estimate using a-priori state estimate
   %K = P*H'*inv(H*P*H'+R); % Kalman gain
        K1 = P([4,5],([4,5]))*inv(P([4,5],([4,5]))+R([4,5],([4,5]))); %H = eye(3)
   %X = X + K*(Z - Z_e); % a-posteriori state estimate
        dZ = Z - Z_e;
        X([4,5]) = X([4,5]) + K1*dZ; % a-posteriori state estimate
   
   %P = (eye(3) - K*H)*P;
    
        P([4,5],([4,5])) = (eye(2) - K1)*P([4,5],([4,5]));
end


function dist = rel_dist_xy(ref_xy,pt_xy)
% This function computes relative distances between given reference point, ref_xy, and positions, p_xy. 
% ref_xy = [x0,y0];
% pt_xy = [x,y];

temp = (pt_xy(:,1)-ref_xy(1)).^2 + (pt_xy(:,2)-ref_xy(2)).^2;
dist = temp.^0.5;

== matlab function bus_roadtest_v3/Flag_management/State management/static_object_judge ==
  settings: updateMethod=DISCRETE
  data: ACC_cmd input; overtake_flag output; Idle_flag input; V2X_Phase input; overtake_over input
function overtake_flag  = fcn(ACC_cmd,Idle_flag,V2X_Phase,overtake_over)

persistent count overtake_state
if isempty(count)
    count = 0;
    overtake_state = 0;
end

if ACC_cmd<2
    count = count+1;
else
    count = 0;
end
if Idle_flag==1 || V2X_Phase==1 || V2X_Phase==3
    count = 0;
end

if count>800 && Idle_flag==0 && (V2X_Phase~=1 && V2X_Phase~=3)
    overtake_state = 1;
end
if overtake_over==1
    overtake_state = 0;
end
overtake_flag = overtake_state;

== matlab function bus_roadtest_v3/Speed_profile/Auto & Check/Static_check ==
  data: Speed_cmd input; Speed_fb input; Static_flag output; Throttle_cmd input
function Static_flag = fcn(Speed_cmd, Speed_fb, Throttle_cmd)

% Static Flag check

if Speed_cmd<0.5 && Throttle_cmd <0.5 && Speed_fb<3
    Static_flag = 1;
else
    Static_flag = 0;
end

% Using condition "Speed_fb < 3" to prevent vehicle from sliding

== matlab function bus_roadtest_v3/Data_RX/OBU/ENU2SLAM ==
  data: Front_Car_x input; Front_Car_SLAM_x output; Front_Car_y input; Front_Car_z input; R input; T input; Front_Car_SLAM_y output; Front_Car_SLAM_z output
function [Front_Car_SLAM_x,Front_Car_SLAM_y,Front_Car_SLAM_z] = fcn(Front_Car_x,Front_Car_y,Front_Car_z,R,T)
R_1 = R(:,1:3);
R_2 = R(:,4:6);
R_3 = R(:,7:9);
R_4 = R(:,10:12);
R_5 = R(:,13:15);

T_1 = T(:,1);
T_2 = T(:,2);
T_3 = T(:,3);
T_4 = T(:,4);
T_5 = T(:,5);

if Front_Car_x <= 0
    R_final = R_1;
    T_final = T_1;
elseif Front_Car_x > 0 && Front_Car_x <= 100
    R_final = R_2;
    T_final = T_2;
elseif Front_Car_x > 100 && Front_Car_x <= 225
    R_final = R_3;
    T_final = T_3;
elseif Front_Car_x > 225 && Front_Car_x <= 350
    R_final = R_4;
    T_final = T_4;
else
    R_final = R_5;
    T_final = T_5;
end

% R_final = R;
% T_final = T;

Car_SLAM_xyz = R_final*[Front_Car_x;Front_Car_y;Front_Car_z] + T_final ;

Front_Car_SLAM_x = Car_SLAM_xyz(1);
Front_Car_SLAM_y = Car_SLAM_xyz(2);
Front_Car_SLAM_z = Car_SLAM_xyz(3);

== matlab function bus_roadtest_v3/Data_RX/Xavier/Filter/MATLAB Function ==
  data: GF input; GF_filtered output; GF_last input
function GF_filtered  = fcn(GF,GF_last)
persistent count
if isempty(count)
    count = 0;
end

if (GF_last-GF) > 200 && count<20
    GF_filtered = GF_last;
    count = count+1;
else
    GF_filtered = GF;
    count = 0;
end

== matlab function bus_roadtest_v3/Positioning_module/ITRI_MM/UKF_Only/SLAM_Generate_sigma_pt_UKF ==
  data: IC_X input; X_AUG output; IC_P input; n input; gamma input
function X_AUG = fcn(IC_X,IC_P,n,gamma)
%#codegen
x0  = IC_X(:,1);
p0 = blkdiag(IC_P(:,1:5));
[p_sqrt,q]= chol(p0);
x_aug=zeros(5,11);

%% model 1
if q ~= 0; % p0 is not positive definite
%     disp('p0 is not positive definite');
    %Reset the covariance matrix by extracting the diagonal of original
    %covariance matrix p0 and check if any element is close to 0, which
    %can cause matrix singularity problem!
    temp_dia = abs(diag(p0));
    indcheck = find(temp_dia(:)<10^-10);
    if ~isempty(indcheck)
        temp_dia(indcheck) = 10^-10;
    end
    %p0 =diag(abs(diag(p0)));
    p0 = diag(temp_dia);
    
    %disp(p0);
    p_sqrt = chol(p0);
end

%%
p_sqrt = gamma.*(p_sqrt');

x_aug(:,1) = x0; %i = 0

for i = 1:n
    x_aug(:,i+1) = x0 + p_sqrt(:,i);
end

for i = 1:n
    x_aug(:,n+1+i) = x0 - p_sqrt(:,i);
end
X_AUG=[x_aug];
